simulink library "AEMS_Standard_Library"  (R2016b)
settings: Solver=ode45  StartTime=0.0  StopTime=10.0  RelTol=1e-3
undefined symbols (not defined in the file or in its folder): BkPY, carto, Cbx_extegr, Cbx_lpegrsys, Cbx_portegr, Cnx_bnk_nr_conf, Cnx_cyl_nr_conf, ConfigManagement, configuration_management, Cxx_dcm_io_tmr_end_xxxx, Cxx_dcm_rt_tmr_end, Cxx_DID_xxxx_IO_max, Cxx_DID_xxxx_IO_min, Cxx_egrhsofs, Cxx_vmaniegi, DEM_DEBOUNCE_FREEZE, DEM_DTR_CTL_INVISIBLE, DEM_DTR_CTL_NORMAL, Dem_DtrId2_XXX, Dem_DtrId3_XXX, Dem_DtrId4_XXX, Dem_DtrId5_XXX, Dem_DtrId6_XXX, Dem_DtrId7_XXX, Dem_DtrId8_XXX, Dem_DtrId9_XXX, Dem_DtrId_XXX, Dem_EnableConditionId2_XXX, Dem_EnableConditionId3_XXX, Dem_EnableConditionId4_XXX, Dem_EnableConditionId5_XXX, Dem_EnableConditionId6_XXX, Dem_EnableConditionId7_XXX, Dem_EnableConditionId8_XXX, Dem_EnableConditionId_XXX, Dem_EventId, Dem_EventId2_XXX, Dem_EventId3_XXX, Dem_EventId4_XXX, Dem_EventId5_XXX, Dem_EventId6_XXX, Dem_EventId7_XXX, Dem_EventId8_XXX, Dem_EventId9_XXX, Dem_EventId_Device_Faulttype, Dem_EventId_XXX, DEM_IUMPR_GENERAL_DENOMINATOR, DEM_OPCYC_IGNITION, Dem_RatioId2_XXX, Dem_RatioId3_XXX, Dem_RatioId4_XXX, Dem_RatioId5_XXX, Dem_RatioId6_XXX, Dem_RatioId7_XXX, Dem_RatioId8_XXX, Dem_RatioId_XXX, Dem_StorageConditionId2_XXX, Dem_StorageConditionId3_XXX, Dem_StorageConditionId4_XXX, Dem_StorageConditionId5_XXX ... (+65)
libraries: AEMS_Standard_Library x477, simulink x2
(part 20 of 39)

== system AEMS_Standard_Library/SPECIFIC/AEMS_SUPPLIER_CALL_PHI_MIN_POST ==
  Data Store Read : DataStoreRead  DataStoreName=Supplier_Call_Phi_Min
      settings: AttributesFormatString=<tsample=%<sampleTime>>
  Vxx_fms_phi_min_post : Outport
  wires:
  Data Store Read/1 -> Vxx_fms_phi_min_post/1

== system AEMS_Standard_Library/SPECIFIC/AEMS_SUPPLIER_CALL_QBA_TQI_MAX_LIM ==
  Tqi_raw_wio_qba : Inport
  Tqi_sp : Inport  Port=2
  DataTypeConversion : DataTypeConversion
  Supplier_Call_QBA_TQI_MAX_LIM : DataStoreRead  DataStoreName=Supplier_Call_QBA_TQI_MAX_LIM
      settings: AttributesFormatString=<tsample=%<sampleTime>>
  Terminator : Terminator
  Terminator1 : Terminator
  Tqi_max_lim_qba : Outport  InitialOutput=0
  wires:
  Tqi_sp/1 -> Terminator1/1
  Tqi_raw_wio_qba/1 -> Terminator/1
  Supplier_Call_QBA_TQI_MAX_LIM/1 -> DataTypeConversion/1
  DataTypeConversion/1 -> Tqi_max_lim_qba/1

== system AEMS_Standard_Library/SPECIFIC/AEMS_SUPPLIER_CALL_SEPA_MIN_AFTR ==
  Data Store Read : DataStoreRead  DataStoreName=Supplier_Call_Sepa_Main_Af_Po
      settings: AttributesFormatString=<tsample=%<sampleTime>>
  Vxx_fms_sep_min_aftr : Outport
  wires:
  Data Store Read/1 -> Vxx_fms_sep_min_aftr/1

== system AEMS_Standard_Library/SPECIFIC/AEMS_SUPPLIER_CALL_SEPA_MIN_LPOS ==
  Data Store Read : DataStoreRead  DataStoreName=Supplier_Call_Sepa_Po_Lpost
      settings: AttributesFormatString=<tsample=%<sampleTime>>
  Vxx_fms_sep_min_lpos : Outport
  wires:
  Data Store Read/1 -> Vxx_fms_sep_min_lpos/1

== system AEMS_Standard_Library/SPECIFIC/AEMS_SUPPLIER_CALL_SEPA_MIN_LPOS2_2SL ==
  Data Store Read : DataStoreRead  DataStoreName=Supplier_Call_Sepa_Lpost1_Lpost2
      settings: AttributesFormatString=<tsample=%<sampleTime>>
  Vxx_fms_sep_min_lpos2_2sl : Outport
  wires:
  Data Store Read/1 -> Vxx_fms_sep_min_lpos2_2sl/1

== system AEMS_Standard_Library/SPECIFIC/AEMS_SUPPLIER_CALL_SEPA_MIN_LPOS2_3SL ==
  Data Store Read : DataStoreRead  DataStoreName=Supplier_Call_Sepa_Lpost1_Lpost2
      settings: AttributesFormatString=<tsample=%<sampleTime>>
  Vxx_fms_sep_min_lpos2_3sl : Outport
  wires:
  Data Store Read/1 -> Vxx_fms_sep_min_lpos2_3sl/1

== system AEMS_Standard_Library/SPECIFIC/AEMS_SUPPLIER_CALL_SEPA_MIN_LPOS2_4SL ==
  Data Store Read : DataStoreRead  DataStoreName=Supplier_Call_Sepa_Lpost1_Lpost2
      settings: AttributesFormatString=<tsample=%<sampleTime>>
  Vxx_fms_sep_min_lpos2_4sl : Outport
  wires:
  Data Store Read/1 -> Vxx_fms_sep_min_lpos2_4sl/1

== system AEMS_Standard_Library/SPECIFIC/AEMS_SUPPLIER_CALL_SEPA_MIN_LPOS3_3SL ==
  Data Store Read : DataStoreRead  DataStoreName=Supplier_Call_Sepa_Lpost1_Lpost2
      settings: AttributesFormatString=<tsample=%<sampleTime>>
  Vxx_fms_sep_min_lpos3_3sl : Outport
  wires:
  Data Store Read/1 -> Vxx_fms_sep_min_lpos3_3sl/1

== system AEMS_Standard_Library/SPECIFIC/AEMS_SUPPLIER_CALL_SEPA_MIN_LPOS3_4SL ==
  Data Store Read : DataStoreRead  DataStoreName=Supplier_Call_Sepa_Lpost1_Lpost2
      settings: AttributesFormatString=<tsample=%<sampleTime>>
  Vxx_fms_sep_min_lpos3_4sl : Outport
  wires:
  Data Store Read/1 -> Vxx_fms_sep_min_lpos3_4sl/1

== system AEMS_Standard_Library/SPECIFIC/AEMS_SUPPLIER_CALL_SEPA_MIN_LPOS4_4SL ==
  Data Store Read : DataStoreRead  DataStoreName=Supplier_Call_Sepa_Lpost1_Lpost2
      settings: AttributesFormatString=<tsample=%<sampleTime>>
  Vxx_fms_sep_min_lpos4_4sl : Outport
  wires:
  Data Store Read/1 -> Vxx_fms_sep_min_lpos4_4sl/1

== system AEMS_Standard_Library/SPECIFIC/AEMS_SUPPLIER_CALL_SEPA_MIN_NXT_CYL ==
  Data Store Read : DataStoreRead  DataStoreName=Supplier_Call_Sepa_Lpost_Pinj
      settings: AttributesFormatString=<tsample=%<sampleTime>>
  Vxx_fms_t_min_nxt_cyl : Outport
  wires:
  Data Store Read/1 -> Vxx_fms_t_min_nxt_cyl/1

== system AEMS_Standard_Library/SPECIFIC/AEMS_SUPPLIER_CALL_SEPA_MIN_NXT_CYL_LPOST2 ==
  Data Store Read : DataStoreRead  DataStoreName=Supplier_Call_Sepa_Lpost_Pinj
      settings: AttributesFormatString=<tsample=%<sampleTime>>
  Vxx_fms_t_min_nxt_cyl_lpos2 : Outport
  wires:
  Data Store Read/1 -> Vxx_fms_t_min_nxt_cyl_lpos2/1

== system AEMS_Standard_Library/SPECIFIC/AEMS_SUPPLIER_CALL_SEPA_MIN_NXT_CYL_LPOST3 ==
  Data Store Read : DataStoreRead  DataStoreName=Supplier_Call_Sepa_Lpost_Pinj
      settings: AttributesFormatString=<tsample=%<sampleTime>>
  Vxx_fms_t_min_nxt_cyl_lpos3 : Outport
  wires:
  Data Store Read/1 -> Vxx_fms_t_min_nxt_cyl_lpos3/1

== system AEMS_Standard_Library/SPECIFIC/AEMS_SUPPLIER_CALL_SEPA_MIN_NXT_CYL_LPOST4 ==
  Data Store Read : DataStoreRead  DataStoreName=Supplier_Call_Sepa_Lpost_Pinj
      settings: AttributesFormatString=<tsample=%<sampleTime>>
  Vxx_fms_t_min_nxt_cyl_lpos4 : Outport
  wires:
  Data Store Read/1 -> Vxx_fms_t_min_nxt_cyl_lpos4/1

== system AEMS_Standard_Library/SPECIFIC/AEMS_SUPPLIER_CALL_SEPA_MIN_PINJ1 ==
  Data Store Read : DataStoreRead  DataStoreName=Supplier_Call_Sepa_P1_P2
      settings: AttributesFormatString=<tsample=%<sampleTime>>
  Vxx_fms_tp1_min : Outport
  wires:
  Data Store Read/1 -> Vxx_fms_tp1_min/1

== system AEMS_Standard_Library/SPECIFIC/AEMS_SUPPLIER_CALL_SEPA_MIN_PINJ2 ==
  Data Store Read : DataStoreRead  DataStoreName=Supplier_Call_Sepa_P2_P3
      settings: AttributesFormatString=<tsample=%<sampleTime>>
  Vxx_fms_tp2_min : Outport
  wires:
  Data Store Read/1 -> Vxx_fms_tp2_min/1

== system AEMS_Standard_Library/SPECIFIC/AEMS_SUPPLIER_CALL_SEPA_MIN_PINJ3 ==
  Data Store Read : DataStoreRead  DataStoreName=Supplier_Call_Sepa_P3_P4
      settings: AttributesFormatString=<tsample=%<sampleTime>>
  Vxx_fms_tp3_min : Outport
  wires:
  Data Store Read/1 -> Vxx_fms_tp3_min/1

== system AEMS_Standard_Library/SPECIFIC/AEMS_SUPPLIER_CALL_SEPA_MIN_PINJ4 ==
  Data Store Read : DataStoreRead  DataStoreName=Supplier_Call_Sepa_Pinj_Main
      settings: AttributesFormatString=<tsample=%<sampleTime>>
  Vxx_fms_tp4_min : Outport
  wires:
  Data Store Read/1 -> Vxx_fms_tp4_min/1

== system AEMS_Standard_Library/SPECIFIC/AEMS_SUPPLIER_CALL_SEPA_MIN_POST ==
  Data Store Read : DataStoreRead  DataStoreName=Supplier_Call_Sepa_Main_Af_Po
      settings: AttributesFormatString=<tsample=%<sampleTime>>
  Vxx_fms_sep_min_post : Outport
  wires:
  Data Store Read/1 -> Vxx_fms_sep_min_post/1

== system AEMS_Standard_Library/SPECIFIC/AEMS_SUPPLIER_CALL_SEPERATION_MIN_TIME ==
  note: Each block will be translated into code C by this way:
      | Output=Supplier call API Name(Splitnum);
      | Example for Supplier_Call_Sepa_min_post1, corresponding output variable is
      | Vxx_fms_sep_min_post1= Supplier_Call_Sepa_min_post1(1);
  note: Splitnum
  DataTypeConversion : DataTypeConversion
  Data_Store_Read : DataStoreRead  DataStoreName=Supplier_Call_Sepa_min_post2
  Splitnum : Constant  Value=3  OutDataTypeStr=uint8
  Terminator1 : Terminator
  Vxx_fms_sep_min_post2_3sl : Outport  InitialOutput=0
  wires:
  Splitnum/1 -> Terminator1/1
  Data_Store_Read/1 -> DataTypeConversion/1
  DataTypeConversion/1 -> Vxx_fms_sep_min_post2_3sl/1

== system AEMS_Standard_Library/SPECIFIC/AEMS_SUPPLIER_CALL_TI_MINI_OK_AFTR ==
  Data Store Read : DataStoreRead  DataStoreName=Supplier_call_ti_mini_ok_aftr
      settings: AttributesFormatString=<tsample=%<sampleTime>>
  Vbx_fms_ti_aftr_min_ok : Outport  InitialOutput=0
  wires:
  Data Store Read/1 -> Vbx_fms_ti_aftr_min_ok/1

== system AEMS_Standard_Library/SPECIFIC/AEMS_SUPPLIER_CALL_TI_MINI_OK_LPOS ==
  Data Store Read : DataStoreRead  DataStoreName=Supplier_call_ti_mini_ok_lpos
      settings: AttributesFormatString=<tsample=%<sampleTime>>
  Vbx_fms_ti_lpos_min_ok : Outport  InitialOutput=0
  wires:
  Data Store Read/1 -> Vbx_fms_ti_lpos_min_ok/1

== system AEMS_Standard_Library/SPECIFIC/AEMS_SUPPLIER_CALL_TI_MINI_OK_LPOS1_2SL ==
  Data Store Read : DataStoreRead  DataStoreName=Supplier_call_ti_mini_ok_lpos1
      settings: AttributesFormatString=<tsample=%<sampleTime>>
  Vbx_fms_ti_lpos1_min_ok_2sl : Outport  InitialOutput=0
  wires:
  Data Store Read/1 -> Vbx_fms_ti_lpos1_min_ok_2sl/1

== system AEMS_Standard_Library/SPECIFIC/AEMS_SUPPLIER_CALL_TI_MINI_OK_LPOS1_3SL ==
  Data Store Read : DataStoreRead  DataStoreName=Supplier_call_ti_mini_ok_lpos1
      settings: AttributesFormatString=<tsample=%<sampleTime>>
  Vbx_fms_ti_lpos1_min_ok_3sl : Outport  InitialOutput=0
  wires:
  Data Store Read/1 -> Vbx_fms_ti_lpos1_min_ok_3sl/1

== system AEMS_Standard_Library/SPECIFIC/AEMS_SUPPLIER_CALL_TI_MINI_OK_LPOS1_4SL ==
  Data Store Read : DataStoreRead  DataStoreName=Supplier_call_ti_mini_ok_lpos1
      settings: AttributesFormatString=<tsample=%<sampleTime>>
  Vbx_fms_ti_lpos1_min_ok_4sl : Outport  InitialOutput=0
  wires:
  Data Store Read/1 -> Vbx_fms_ti_lpos1_min_ok_4sl/1

== system AEMS_Standard_Library/SPECIFIC/AEMS_SUPPLIER_CALL_TI_MINI_OK_LPOS2_2SL ==
  Data Store Read : DataStoreRead  DataStoreName=Supplier_call_ti_mini_ok_lpos2
      settings: AttributesFormatString=<tsample=%<sampleTime>>
  Vbx_fms_ti_lpos2_min_ok_2sl : Outport  InitialOutput=0
  wires:
  Data Store Read/1 -> Vbx_fms_ti_lpos2_min_ok_2sl/1

== system AEMS_Standard_Library/SPECIFIC/AEMS_SUPPLIER_CALL_TI_MINI_OK_LPOS2_3SL ==
  Data Store Read : DataStoreRead  DataStoreName=Supplier_call_ti_mini_ok_lpos2
      settings: AttributesFormatString=<tsample=%<sampleTime>>
  Vbx_fms_ti_lpos2_min_ok_3sl : Outport  InitialOutput=0
  wires:
  Data Store Read/1 -> Vbx_fms_ti_lpos2_min_ok_3sl/1

== system AEMS_Standard_Library/SPECIFIC/AEMS_SUPPLIER_CALL_TI_MINI_OK_LPOS2_4SL ==
  Data Store Read : DataStoreRead  DataStoreName=Supplier_call_ti_mini_ok_lpos3
      settings: AttributesFormatString=<tsample=%<sampleTime>>
  Vbx_fms_ti_lpos2_min_ok_4sl : Outport  InitialOutput=0
  wires:
  Data Store Read/1 -> Vbx_fms_ti_lpos2_min_ok_4sl/1

== system AEMS_Standard_Library/SPECIFIC/AEMS_SUPPLIER_CALL_TI_MINI_OK_LPOS3_3SL ==
  Data Store Read : DataStoreRead  DataStoreName=Supplier_call_ti_mini_ok_lpos3
      settings: AttributesFormatString=<tsample=%<sampleTime>>
  Vbx_fms_ti_lpos3_min_ok_3sl : Outport  InitialOutput=0
  wires:
  Data Store Read/1 -> Vbx_fms_ti_lpos3_min_ok_3sl/1

== system AEMS_Standard_Library/SPECIFIC/AEMS_SUPPLIER_CALL_TI_MINI_OK_LPOS3_4SL ==
  Data Store Read : DataStoreRead  DataStoreName=Supplier_call_ti_mini_ok_lpos2
      settings: AttributesFormatString=<tsample=%<sampleTime>>
  Vbx_fms_ti_lpos3_min_ok_4sl : Outport  InitialOutput=0
  wires:
  Data Store Read/1 -> Vbx_fms_ti_lpos3_min_ok_4sl/1

== system AEMS_Standard_Library/SPECIFIC/AEMS_SUPPLIER_CALL_TI_MINI_OK_LPOS4_4SL ==
  Data Store Read : DataStoreRead  DataStoreName=Supplier_call_ti_mini_ok_lpos4
      settings: AttributesFormatString=<tsample=%<sampleTime>>
  Vbx_fms_ti_lpos4_min_ok_4sl : Outport  InitialOutput=0
  wires:
  Data Store Read/1 -> Vbx_fms_ti_lpos4_min_ok_4sl/1

== system AEMS_Standard_Library/SPECIFIC/AEMS_SUPPLIER_CALL_TI_MINI_OK_MAIN ==
  Data Store Read : DataStoreRead  DataStoreName=Supplier_call_ti_mini_ok_main
      settings: AttributesFormatString=<tsample=%<sampleTime>>
  Vbx_fms_ti_main_min_ok : Outport  InitialOutput=0
  wires:
  Data Store Read/1 -> Vbx_fms_ti_main_min_ok/1

== system AEMS_Standard_Library/SPECIFIC/AEMS_SUPPLIER_CALL_TI_MINI_OK_PINJ1 ==
  Data Store Read : DataStoreRead  DataStoreName=Supplier_call_ti_mini_ok_pinj1
      settings: AttributesFormatString=<tsample=%<sampleTime>>
  Vbx_fms_ti_pinj1_min_ok : Outport  InitialOutput=0
  wires:
  Data Store Read/1 -> Vbx_fms_ti_pinj1_min_ok/1

== system AEMS_Standard_Library/SPECIFIC/AEMS_SUPPLIER_CALL_TI_MINI_OK_PINJ2 ==
  Data Store Read : DataStoreRead  DataStoreName=Supplier_call_ti_mini_ok_pinj2
      settings: AttributesFormatString=<tsample=%<sampleTime>>
  Vbx_fms_ti_pinj2_min_ok : Outport  InitialOutput=0
  wires:
  Data Store Read/1 -> Vbx_fms_ti_pinj2_min_ok/1

== system AEMS_Standard_Library/SPECIFIC/AEMS_SUPPLIER_CALL_TI_MINI_OK_PINJ3 ==
  Data Store Read : DataStoreRead  DataStoreName=Supplier_call_ti_mini_ok_pinj3
      settings: AttributesFormatString=<tsample=%<sampleTime>>
  Vbx_fms_ti_pinj3_min_ok : Outport  InitialOutput=0
  wires:
  Data Store Read/1 -> Vbx_fms_ti_pinj3_min_ok/1

== system AEMS_Standard_Library/SPECIFIC/AEMS_SUPPLIER_CALL_TI_MINI_OK_PINJ4 ==
  DataStoreRead : DataStoreRead  DataStoreName=Supplier_call_ti_mini_ok_pinj4
      settings: AttributesFormatString=<tsample=%<sampleTime>>
  Vbx_fms_ti_pinj4_min_ok : Outport  InitialOutput=0
  wires:
  DataStoreRead/1 -> Vbx_fms_ti_pinj4_min_ok/1

== system AEMS_Standard_Library/SPECIFIC/AEMS_SUPPLIER_CALL_TI_MINI_OK_POST ==
  Data Store Read : DataStoreRead  DataStoreName=Supplier_call_ti_mini_ok_post
      settings: AttributesFormatString=<tsample=%<sampleTime>>
  Vbx_fms_ti_post_min_ok : Outport  InitialOutput=0
  wires:
  Data Store Read/1 -> Vbx_fms_ti_post_min_ok/1

== system AEMS_Standard_Library/SPECIFIC/AEMS_SUPPLIER_CALL_TI_MIN_OK ==
  note: Coding information: This block is to call Supplier call API.
      | Each block will be translated into code C by this way:
      | Output=Supplier call API Name(Splitnum);
      | Example for Supplier_Call_Ti_mini_post2_ok, corresponding output variable is
      | Vbx_fms_ti_min_post2_2sl_ok= Supplier_Call_Ti_mini_post2_ok(2);
  note: Splitnum
  DataTypeConversion : DataTypeConversion
  Data_Store_Read : DataStoreRead  DataStoreName=Supplier_Call_Ti_mini_post2_ok
      settings: AttributesFormatString=<tsample=%<sampleTime>>
  Splitnum : Constant  Value=2  OutDataTypeStr=uint8
  Terminator1 : Terminator
  Vbx_fms_ti_min_post2_2sl_ok : Outport  InitialOutput=0
  wires:
  DataTypeConversion/1 -> Vbx_fms_ti_min_post2_2sl_ok/1
  Splitnum/1 -> Terminator1/1
  Data_Store_Read/1 -> DataTypeConversion/1

== system AEMS_Standard_Library/SPECIFIC/AEMS_SlopeSwitchExtern ==
  Switch_Cmd : Inport
  Pos_Slope : Inport  Port=2
  Neg_Slope : Inport  Port=3
  Input : Inport  Port=4
  dT : Inport  Port=5
  Estimate_transition_time : Subsystem
  Product : Product  OutDataTypeStr=Inherit: Inherit via back propagation  RndMeth=Zero
  Product1 : Product  OutDataTypeStr=Inherit: Inherit via back propagation  RndMeth=Zero
  Saturation : Saturate  UpperLimit=1  LowerLimit=0  RndMeth=Zero
      settings: AttributesFormatString=<limits=%<UpperLimit>/%<LowerLimit>>
  Selector : Selector  IndexMode=Zero-based  InputPortWidth=LimitDimInputs  IndexOptions=Index vector (port)  Indices=[1 3]  OutputSizes=1
  Signal_Change_Compute : Subsystem
  Slope_On_Block : Subsystem
  Slope_On_Compute : Subsystem
  Switch2 : Switch  Criteria=u2 ~= 0  RndMeth=Zero  SaturateOnIntegerOverflow=on  InputSameDT=on
      settings: AttributesFormatString=Criteria=%<Criteria>
  UnitDelay1 : UnitDelay  InitialCondition=false  SampleTime=-1
      settings: AttributesFormatString=<initial=%<InitialCondition>>
  UnitDelay2 : UnitDelay  SampleTime=-1
      settings: AttributesFormatString=<initial=%<InitialCondition>>
  Output : Outport
  Slope_On : Outport  Port=2
  Rem_Transition_Time : Outport  Port=3
  wires:
  Neg_Slope/1 -> Product1/2, Estimate_transition_time/4(Neg_Slope)
  Selector/1 -> Switch2/3, Estimate_transition_time/1(Input), Slope_On_Block/2(Input)
  Pos_Slope/1 -> Product/2, Estimate_transition_time/3(Pos_Slope)
  Slope_On_Block/1(Output_Not_Equals_Input) -> UnitDelay1/1
  Switch2/1 -> UnitDelay2/1, Estimate_transition_time/2(Output), Output/1
  Slope_On_Compute/1(Slope_On) -> Switch2/2, Slope_On_Block/Enable, Slope_On/1  "Slope_On"
  Slope_On_Block/2(Output) -> Switch2/1
  UnitDelay1/1 -> Slope_On_Compute/2(Output_Not_Equals_Input)
  Switch_Cmd/1 -> Saturation/1
  UnitDelay2/1 -> Slope_On_Block/5(Prev_Output)
  Product/1 -> Slope_On_Block/3(Pos_Slope)
  Product1/1 -> Slope_On_Block/4(Neg_Slope)
  Signal_Change_Compute/1(Signal_Change) -> Slope_On_Compute/1(Signal_Change), Slope_On_Block/1(Signal_Change)
  dT/1 -> Product/1, Product1/1
  Estimate_transition_time/1(Rem_Transition_Time) -> Rem_Transition_Time/1
  Input/1 -> Selector/1
  Saturation/1 -> Selector/2, Signal_Change_Compute/1(Switch_Cmd)

== system AEMS_Standard_Library/SPECIFIC/AEMS_UL_INTERP ==
  input_of_ratio_1 : Inport
      settings: AttributesFormatString=<tsample=%<sampleTime>>
  interpolate_ratio : Inport  Port=2
      settings: AttributesFormatString=<tsample=%<sampleTime>>
  input_of_ratio_0 : Inport  Port=3
      settings: AttributesFormatString=<tsample=%<sampleTime>>
  Constant1 : Constant  OutDataTypeStr=Inherit: Inherit via back propagation
  Product : Product  OutDataTypeStr=Inherit: Inherit via back propagation  RndMeth=Zero
  Product1 : Product  OutDataTypeStr=Inherit: Inherit via back propagation  RndMeth=Zero
  Saturation : Saturate  UpperLimit=1  LowerLimit=0
      settings: AttributesFormatString=<limits=%<upperlimit> / %<lowerlimit>>
  Sum : Sum  Inputs=-+  SaturateOnIntegerOverflow=on  InputSameDT=on
  Sum1 : Sum  SaturateOnIntegerOverflow=on  InputSameDT=on
  output : Outport
  wires:
  Sum1/1 -> output/1
  Constant1/1 -> Sum/2
  input_of_ratio_0/1 -> Product1/2
  Product1/1 -> Sum1/2
  Product/1 -> Sum1/1
  Sum/1 -> Product1/1
  interpolate_ratio/1 -> Saturation/1
  input_of_ratio_1/1 -> Product/1
  Saturation/1 -> Product/2, Sum/1

== system AEMS_Standard_Library/SUB/AEMS_CONVERT_BUFFER_TO_FLP ==
  note: Scalar Value in FXP
  note: Value_FLP
  note: Conversion from FXP to FLP
      |
      | Data converted from FXP to FLP using Resolution and Offset of variable DID
  note: ERRORCode: Retrun status of Error Code
      |
      | Data written by DCM in array form and converted to
      | a scalar by multiplied by factor [1 2^8 2^16 2^24] depend on size of DID
  Buffer : Inport
  Chart1 : Stateflow chart  TreatAsAtomicUnit=on
  Constant : Constant  Value=DID_Datatype  OutDataTypeStr=uint8
  Data Type Conversion : DataTypeConversion
  Mux : Mux  Inputs=3
  Offset : Constant  Value=offset  OutDataTypeStr=Inherit: Inherit via back propagation
  Product1 : Product  OutDataTypeStr=Inherit: Inherit via back propagation  RndMeth=Zero
  Resol : Constant  Value=Resol  OutDataTypeStr=Inherit: Inherit via back propagation
  Sum1 : Sum  OutDataTypeStr=Inherit: Inherit via back propagation  RndMeth=Zero  InputSameDT=on
  Terminator : Terminator
  Value_float : Outport
  wires:
  Mux/1 -> Terminator/1
  Sum1/1 -> Value_float/1, Mux/1
  Product1/1 -> Sum1/1
  Resol/1 -> Product1/2, Mux/3
  Offset/1 -> Sum1/2, Mux/2
  Data Type Conversion/1 -> Product1/1
  Buffer/1 -> Chart1/2(Input_Buff)
  Chart1/1(Fxp_Scalar_Value) -> Data Type Conversion/1
  Constant/1 -> Chart1/1(DataType)

== system AEMS_Standard_Library/SUB/AEMS_CONVERT_BYTE_TO_FLP ==
  note: ERRORCode: Retrun status of Error Code
      |
      | Data written by DCM in array form and converted to
      | a scalar by multiplied by factor [1 2^8 2^16 2^24] depend on size of DID
  note: Conversion from FXP to FLP
      |
      | Data converted from FXP to FLP using Resolution and Offset of variable DID
  note: Value_FLP
  note: Scalar Value in FXP
  Input : Inport
  Chart1 : Stateflow chart  TreatAsAtomicUnit=on
  Constant : Constant  Value=DID_Datatype  OutDataTypeStr=uint8
  Data Type Conversion : DataTypeConversion
  Mux : Mux  Inputs=3
  Offset : Constant  Value=offset  OutDataTypeStr=Inherit: Inherit via back propagation
  Product1 : Product  OutDataTypeStr=Inherit: Inherit via back propagation  RndMeth=Zero
  Resol : Constant  Value=Resol  OutDataTypeStr=Inherit: Inherit via back propagation
  Sum1 : Sum  OutDataTypeStr=Inherit: Inherit via back propagation  RndMeth=Zero  InputSameDT=on
  Terminator : Terminator
  Value_float : Outport
  wires:
  Constant/1 -> Chart1/1(DataType)
  Chart1/1(Fxp_Scalar_Value) -> Data Type Conversion/1
  Input/1 -> Chart1/2(Input)
  Data Type Conversion/1 -> Product1/1
  Offset/1 -> Mux/2, Sum1/2
  Resol/1 -> Mux/3, Product1/2
  Product1/1 -> Sum1/1
  Sum1/1 -> Mux/1, Value_float/1
  Mux/1 -> Terminator/1

== system AEMS_Standard_Library/SUB/AEMS_DEM_COUNTERBASEDDEBOUNCE ==
  conditionfulfilled : Inport
  prefailed : Inport  Port=2
  prepassed : Inport  Port=3
  reseteventdebounce : Inport  Port=4
  DemDebounceBehavior : Inport  Port=5
  DemCounterFailedThreshold : Inport  Port=6
  DemCounterIncrementStepSize : Inport  Port=7
  DemCounterJumpUp : Inport  Port=8
  DemCounterJumpUpValue : Inport  Port=9
  DemCounterPassedThreshold : Inport  Port=10
  DemCounterDecrementStepSize : Inport  Port=11
  DemCounterJumpDown : Inport  Port=12
  DemCounterJumpDownValue : Inport  Port=13
  Counter_Debounce : Subsystem
  Dem_SetEventStatus_Call : Subsystem  TreatAsAtomicUnit=on
  debouncevalue : Outport
  failed : Outport  Port=2
  passed : Outport  Port=3
  wires:
  conditionfulfilled/1 -> Counter_Debounce/1(conditionfulfilled)
  Counter_Debounce/3(passed) -> passed/1
  Counter_Debounce/2(failed) -> failed/1
  reseteventdebounce/1 -> Counter_Debounce/13(reseteventdebounce)
  DemCounterJumpDownValue/1 -> Counter_Debounce/12(jumpdownvalue_with_prepassed)
  DemCounterJumpDown/1 -> Counter_Debounce/11(jumpdown_activation_with_prepassed)
  DemCounterDecrementStepSize/1 -> Counter_Debounce/10(decrementstepsize_for_prepassed)
  DemCounterPassedThreshold/1 -> Counter_Debounce/9(passedthreshold)
  DemCounterJumpUpValue/1 -> Counter_Debounce/8(jumpupvalue_with_prefailed)
  DemCounterJumpUp/1 -> Counter_Debounce/7(jumpup_activation_with_prefailed)
  DemCounterIncrementStepSize/1 -> Counter_Debounce/6(incrementstepsize_for_prefailed)
  Counter_Debounce/5(eventstatus) -> Dem_SetEventStatus_Call/1(event_status)
  DemCounterFailedThreshold/1 -> Counter_Debounce/5(failedthreshold)
  DemDebounceBehavior/1 -> Counter_Debounce/4(behavior)
  prefailed/1 -> Counter_Debounce/2(prefailed)
  prepassed/1 -> Counter_Debounce/3(prepassed)
  Counter_Debounce/1(debouncevalue) -> debouncevalue/1
  Counter_Debounce/4(call_seteventstatus) -> Dem_SetEventStatus_Call/Enable

== system AEMS_Standard_Library/SUB/AEMS_DEM_COUNTER_BASED_DEBOUNCE_1D ==
  note: DemDebounceBehavior
  flag_set : Inport
  conditionfulfilled : Inport  Port=2
  prefailed : Inport  Port=3
  prepassed : Inport  Port=4
  reseteventdebounce : Inport  Port=5
  AEMS_DEM_COUNTER_BASED_DEBOUNCE_CALL : Subsystem
  DemCounterDecrementStepSize : Constant  Value=DemCounterDecrementStepSize
  DemCounterFailedThreshold : Constant  Value=DemCounterFailedThreshold
  DemCounterIncrementStepSize : Constant  Value=DemCounterIncrementStepSize
  DemCounterJumpDown : Constant  Value=DemCounterJumpDown
  DemCounterJumpDownValue : Constant  Value=DemCounterJumpDownValue
  DemCounterJumpUp : Constant  Value=DemCounterJumpUp
  DemCounterJumpUpValue : Constant  Value=DemCounterJumpUpValue
  DemCounterPassedThreshold : Constant  Value=DemCounterPassedThreshold
  DemDebounceBehavior : Constant  Value=0  OutDataTypeStr=uint8
  debouncevalue : Outport
  failed : Outport  Port=2
  passed : Outport  Port=3
  wires:
  flag_set/1 -> AEMS_DEM_COUNTER_BASED_DEBOUNCE_CALL/Enable
  AEMS_DEM_COUNTER_BASED_DEBOUNCE_CALL/3(passed) -> passed/1
  AEMS_DEM_COUNTER_BASED_DEBOUNCE_CALL/2(failed) -> failed/1
  AEMS_DEM_COUNTER_BASED_DEBOUNCE_CALL/1(debouncevalue) -> debouncevalue/1
  DemCounterJumpDownValue/1 -> AEMS_DEM_COUNTER_BASED_DEBOUNCE_CALL/13(DemCounterJumpDownValue)  "jumpupvalue_with_prefailed"
  DemCounterJumpDown/1 -> AEMS_DEM_COUNTER_BASED_DEBOUNCE_CALL/12(DemCounterJumpDown)  "jumpdown_activation_with_prepassed"
  DemCounterDecrementStepSize/1 -> AEMS_DEM_COUNTER_BASED_DEBOUNCE_CALL/11(DemCounterDecrementStepSize)  "decrementstepsize_for_prepassed"
  DemCounterPassedThreshold/1 -> AEMS_DEM_COUNTER_BASED_DEBOUNCE_CALL/10(DemCounterPassedThreshold)  "passedthreshold"
  DemCounterJumpUpValue/1 -> AEMS_DEM_COUNTER_BASED_DEBOUNCE_CALL/9(DemCounterJumpUpValue)  "jumpupvalue_with_prefailed"
  DemCounterJumpUp/1 -> AEMS_DEM_COUNTER_BASED_DEBOUNCE_CALL/8(DemCounterJumpUp)  "jumpup_activation_with_prefailed"
  DemCounterIncrementStepSize/1 -> AEMS_DEM_COUNTER_BASED_DEBOUNCE_CALL/7(DemCounterIncrementStepSize)  "incrementstepsize_for_prefailed"
  DemCounterFailedThreshold/1 -> AEMS_DEM_COUNTER_BASED_DEBOUNCE_CALL/6(DemCounterFailedThreshold)  "failedthreshold"
  DemDebounceBehavior/1 -> AEMS_DEM_COUNTER_BASED_DEBOUNCE_CALL/5(DemDebounceBehavior)  "behavior"
  reseteventdebounce/1 -> AEMS_DEM_COUNTER_BASED_DEBOUNCE_CALL/4(reseteventdebounce)  "reseteventdebounce"
  prepassed/1 -> AEMS_DEM_COUNTER_BASED_DEBOUNCE_CALL/3(prepassed)  "prepassed"
  prefailed/1 -> AEMS_DEM_COUNTER_BASED_DEBOUNCE_CALL/2(prefailed)  "prefailed"
  conditionfulfilled/1 -> AEMS_DEM_COUNTER_BASED_DEBOUNCE_CALL/1(conditionfulfilled)  "conditionfulfilled"

== system AEMS_Standard_Library/SUB/AEMS_DEM_COUNTER_BASED_DEBOUNCE_2D ==
  note: DemDebounceBehavior
  flag_set : Inport
  conditionfulfilled : Inport  Port=2
  prefailed : Inport  Port=3
  prepassed : Inport  Port=4
  reseteventdebounce : Inport  Port=5
  AEMS_DEM_COUNTER_BASED_DEBOUNCE_CALL1 : Subsystem
  AEMS_DEM_COUNTER_BASED_DEBOUNCE_CALL2 : Subsystem
  DemCounterDecrementStepSize : Constant  Value=DemCounterDecrementStepSize
  DemCounterFailedThreshold : Constant  Value=DemCounterFailedThreshold
  DemCounterIncrementStepSize : Constant  Value=DemCounterIncrementStepSize
  DemCounterJumpDown : Constant  Value=DemCounterJumpDown
  DemCounterJumpDownValue : Constant  Value=DemCounterJumpDownValue
  DemCounterJumpUp : Constant  Value=DemCounterJumpUp
  DemCounterJumpUpValue : Constant  Value=DemCounterJumpUpValue
  DemCounterPassedThreshold : Constant  Value=DemCounterPassedThreshold
  DemDebounceBehavior : Constant  Value=[0,0]  OutDataTypeStr=uint8
  Demux{,1..4} (5 alike) : Demux  Outputs=[1,1]
  Demux{5..13} (9 alike) : Demux  Outputs=2
  Mux : Mux  Inputs=2
  Mux1 : Mux  Inputs=2
  Mux2 : Mux  Inputs=2
  debouncevalue : Outport
  failed : Outport  Port=2
  passed : Outport  Port=3
  wires:
  AEMS_DEM_COUNTER_BASED_DEBOUNCE_CALL2/3(passed) -> Mux/2
  AEMS_DEM_COUNTER_BASED_DEBOUNCE_CALL2/2(failed) -> Mux2/2
  AEMS_DEM_COUNTER_BASED_DEBOUNCE_CALL2/1(debouncevalue) -> Mux1/2
  AEMS_DEM_COUNTER_BASED_DEBOUNCE_CALL1/3(passed) -> Mux/1
  AEMS_DEM_COUNTER_BASED_DEBOUNCE_CALL1/2(failed) -> Mux2/1
  AEMS_DEM_COUNTER_BASED_DEBOUNCE_CALL1/1(debouncevalue) -> Mux1/1
  Mux2/1 -> failed/1
  Mux1/1 -> debouncevalue/1
  Mux/1 -> passed/1
  Demux7/1 -> AEMS_DEM_COUNTER_BASED_DEBOUNCE_CALL1/13(DemCounterJumpDownValue)
  Demux6/1 -> AEMS_DEM_COUNTER_BASED_DEBOUNCE_CALL1/12(DemCounterJumpDown)
  Demux5/1 -> AEMS_DEM_COUNTER_BASED_DEBOUNCE_CALL1/11(DemCounterDecrementStepSize)
  Demux10/1 -> AEMS_DEM_COUNTER_BASED_DEBOUNCE_CALL1/10(DemCounterPassedThreshold)
  Demux9/1 -> AEMS_DEM_COUNTER_BASED_DEBOUNCE_CALL1/9(DemCounterJumpUpValue)
  Demux8/1 -> AEMS_DEM_COUNTER_BASED_DEBOUNCE_CALL1/8(DemCounterJumpUp)
  Demux13/1 -> AEMS_DEM_COUNTER_BASED_DEBOUNCE_CALL1/7(DemCounterIncrementStepSize)
  Demux12/1 -> AEMS_DEM_COUNTER_BASED_DEBOUNCE_CALL1/6(DemCounterFailedThreshold)
  Demux11/1 -> AEMS_DEM_COUNTER_BASED_DEBOUNCE_CALL1/5(DemDebounceBehavior)
  Demux4/1 -> AEMS_DEM_COUNTER_BASED_DEBOUNCE_CALL1/4(reseteventdebounce)
  Demux3/1 -> AEMS_DEM_COUNTER_BASED_DEBOUNCE_CALL1/3(prepassed)
  Demux2/1 -> AEMS_DEM_COUNTER_BASED_DEBOUNCE_CALL1/2(prefailed)
  Demux1/1 -> AEMS_DEM_COUNTER_BASED_DEBOUNCE_CALL1/1(conditionfulfilled)
  Demux/1 -> AEMS_DEM_COUNTER_BASED_DEBOUNCE_CALL1/Enable
  Demux/2 -> AEMS_DEM_COUNTER_BASED_DEBOUNCE_CALL2/Enable
  Demux1/2 -> AEMS_DEM_COUNTER_BASED_DEBOUNCE_CALL2/1(conditionfulfilled)
  Demux2/2 -> AEMS_DEM_COUNTER_BASED_DEBOUNCE_CALL2/2(prefailed)
  Demux3/2 -> AEMS_DEM_COUNTER_BASED_DEBOUNCE_CALL2/3(prepassed)
  Demux4/2 -> AEMS_DEM_COUNTER_BASED_DEBOUNCE_CALL2/4(reseteventdebounce)
  Demux11/2 -> AEMS_DEM_COUNTER_BASED_DEBOUNCE_CALL2/5(DemDebounceBehavior)
  Demux12/2 -> AEMS_DEM_COUNTER_BASED_DEBOUNCE_CALL2/6(DemCounterFailedThreshold)
  Demux13/2 -> AEMS_DEM_COUNTER_BASED_DEBOUNCE_CALL2/7(DemCounterIncrementStepSize)
  Demux8/2 -> AEMS_DEM_COUNTER_BASED_DEBOUNCE_CALL2/8(DemCounterJumpUp)
  Demux9/2 -> AEMS_DEM_COUNTER_BASED_DEBOUNCE_CALL2/9(DemCounterJumpUpValue)
  Demux10/2 -> AEMS_DEM_COUNTER_BASED_DEBOUNCE_CALL2/10(DemCounterPassedThreshold)
  Demux5/2 -> AEMS_DEM_COUNTER_BASED_DEBOUNCE_CALL2/11(DemCounterDecrementStepSize)
  Demux6/2 -> AEMS_DEM_COUNTER_BASED_DEBOUNCE_CALL2/12(DemCounterJumpDown)
  Demux7/2 -> AEMS_DEM_COUNTER_BASED_DEBOUNCE_CALL2/13(DemCounterJumpDownValue)
  DemCounterIncrementStepSize/1 -> Demux13/1  "incrementstepsize_for_prefailed"
  DemCounterFailedThreshold/1 -> Demux12/1  "failedthreshold"
  DemDebounceBehavior/1 -> Demux11/1  "behavior"
  DemCounterPassedThreshold/1 -> Demux10/1  "passedthreshold"
  DemCounterJumpUpValue/1 -> Demux9/1  "jumpupvalue_with_prefailed"
  DemCounterJumpUp/1 -> Demux8/1  "jumpup_activation_with_prefailed"
  DemCounterJumpDownValue/1 -> Demux7/1  "jumpupvalue_with_prefailed"
  DemCounterJumpDown/1 -> Demux6/1  "jumpdown_activation_with_prepassed"
  DemCounterDecrementStepSize/1 -> Demux5/1  "decrementstepsize_for_prepassed"
  reseteventdebounce/1 -> Demux4/1  "reseteventdebounce"
  prepassed/1 -> Demux3/1  "prepassed"
  prefailed/1 -> Demux2/1  "prefailed"
  conditionfulfilled/1 -> Demux1/1  "conditionfulfilled"
  flag_set/1 -> Demux/1

== system AEMS_Standard_Library/SUB/AEMS_DEM_COUNTER_BASED_DEBOUNCE_3D ==
  note: DemDebounceBehavior
  flag_set : Inport
  conditionfulfilled : Inport  Port=2
  prefailed : Inport  Port=3
  prepassed : Inport  Port=4
  reseteventdebounce : Inport  Port=5
  AEMS_DEM_COUNTER_BASED_DEBOUNCE_CALL1 : Subsystem
  AEMS_DEM_COUNTER_BASED_DEBOUNCE_CALL2 : Subsystem
  AEMS_DEM_COUNTER_BASED_DEBOUNCE_CALL3 : Subsystem
  DemCounterDecrementStepSize : Constant  Value=DemCounterDecrementStepSize
  DemCounterFailedThreshold : Constant  Value=DemCounterFailedThreshold
  DemCounterIncrementStepSize : Constant  Value=DemCounterIncrementStepSize
  DemCounterJumpDown : Constant  Value=DemCounterJumpDown
  DemCounterJumpDownValue : Constant  Value=DemCounterJumpDownValue
  DemCounterJumpUp : Constant  Value=DemCounterJumpUp
  DemCounterJumpUpValue : Constant  Value=DemCounterJumpUpValue
  DemCounterPassedThreshold : Constant  Value=DemCounterPassedThreshold
  DemDebounceBehavior : Constant  Value=[0,0,0]  OutDataTypeStr=uint8
  Demux{,1..13} (14 alike) : Demux  Outputs=3
  Mux : Mux  Inputs=3
  Mux1 : Mux  Inputs=3
  Mux2 : Mux  Inputs=3
  debouncevalue : Outport
  failed : Outport  Port=2
  passed : Outport  Port=3
  wires:
  AEMS_DEM_COUNTER_BASED_DEBOUNCE_CALL3/3(passed) -> Mux/3
  AEMS_DEM_COUNTER_BASED_DEBOUNCE_CALL3/2(failed) -> Mux2/3
  AEMS_DEM_COUNTER_BASED_DEBOUNCE_CALL3/1(debouncevalue) -> Mux1/3
  Demux7/3 -> AEMS_DEM_COUNTER_BASED_DEBOUNCE_CALL3/13(DemCounterJumpDownValue)
  Demux6/3 -> AEMS_DEM_COUNTER_BASED_DEBOUNCE_CALL3/12(DemCounterJumpDown)
  Demux5/3 -> AEMS_DEM_COUNTER_BASED_DEBOUNCE_CALL3/11(DemCounterDecrementStepSize)
  Demux10/3 -> AEMS_DEM_COUNTER_BASED_DEBOUNCE_CALL3/10(DemCounterPassedThreshold)
  Demux9/3 -> AEMS_DEM_COUNTER_BASED_DEBOUNCE_CALL3/9(DemCounterJumpUpValue)
  Demux8/3 -> AEMS_DEM_COUNTER_BASED_DEBOUNCE_CALL3/8(DemCounterJumpUp)
  Demux13/3 -> AEMS_DEM_COUNTER_BASED_DEBOUNCE_CALL3/7(DemCounterIncrementStepSize)
  Demux12/3 -> AEMS_DEM_COUNTER_BASED_DEBOUNCE_CALL3/6(DemCounterFailedThreshold)
  Demux11/3 -> AEMS_DEM_COUNTER_BASED_DEBOUNCE_CALL3/5(DemDebounceBehavior)
  Demux4/3 -> AEMS_DEM_COUNTER_BASED_DEBOUNCE_CALL3/4(reseteventdebounce)
  Demux3/3 -> AEMS_DEM_COUNTER_BASED_DEBOUNCE_CALL3/3(prepassed)
  Demux2/3 -> AEMS_DEM_COUNTER_BASED_DEBOUNCE_CALL3/2(prefailed)
  Demux1/3 -> AEMS_DEM_COUNTER_BASED_DEBOUNCE_CALL3/1(conditionfulfilled)
  Demux/3 -> AEMS_DEM_COUNTER_BASED_DEBOUNCE_CALL3/Enable
  AEMS_DEM_COUNTER_BASED_DEBOUNCE_CALL2/3(passed) -> Mux/2
  AEMS_DEM_COUNTER_BASED_DEBOUNCE_CALL2/2(failed) -> Mux2/2
  AEMS_DEM_COUNTER_BASED_DEBOUNCE_CALL2/1(debouncevalue) -> Mux1/2
  AEMS_DEM_COUNTER_BASED_DEBOUNCE_CALL1/3(passed) -> Mux/1
  AEMS_DEM_COUNTER_BASED_DEBOUNCE_CALL1/2(failed) -> Mux2/1
  AEMS_DEM_COUNTER_BASED_DEBOUNCE_CALL1/1(debouncevalue) -> Mux1/1
  Mux2/1 -> failed/1
  Mux1/1 -> debouncevalue/1
  Mux/1 -> passed/1
  Demux7/1 -> AEMS_DEM_COUNTER_BASED_DEBOUNCE_CALL1/13(DemCounterJumpDownValue)
  Demux6/1 -> AEMS_DEM_COUNTER_BASED_DEBOUNCE_CALL1/12(DemCounterJumpDown)
  Demux5/1 -> AEMS_DEM_COUNTER_BASED_DEBOUNCE_CALL1/11(DemCounterDecrementStepSize)
  Demux10/1 -> AEMS_DEM_COUNTER_BASED_DEBOUNCE_CALL1/10(DemCounterPassedThreshold)
  Demux9/1 -> AEMS_DEM_COUNTER_BASED_DEBOUNCE_CALL1/9(DemCounterJumpUpValue)
  Demux8/1 -> AEMS_DEM_COUNTER_BASED_DEBOUNCE_CALL1/8(DemCounterJumpUp)
  Demux13/1 -> AEMS_DEM_COUNTER_BASED_DEBOUNCE_CALL1/7(DemCounterIncrementStepSize)
  Demux12/1 -> AEMS_DEM_COUNTER_BASED_DEBOUNCE_CALL1/6(DemCounterFailedThreshold)
  Demux11/1 -> AEMS_DEM_COUNTER_BASED_DEBOUNCE_CALL1/5(DemDebounceBehavior)
  Demux4/1 -> AEMS_DEM_COUNTER_BASED_DEBOUNCE_CALL1/4(reseteventdebounce)
  Demux3/1 -> AEMS_DEM_COUNTER_BASED_DEBOUNCE_CALL1/3(prepassed)
  Demux2/1 -> AEMS_DEM_COUNTER_BASED_DEBOUNCE_CALL1/2(prefailed)
  Demux1/1 -> AEMS_DEM_COUNTER_BASED_DEBOUNCE_CALL1/1(conditionfulfilled)
  Demux/1 -> AEMS_DEM_COUNTER_BASED_DEBOUNCE_CALL1/Enable
  Demux/2 -> AEMS_DEM_COUNTER_BASED_DEBOUNCE_CALL2/Enable
  Demux1/2 -> AEMS_DEM_COUNTER_BASED_DEBOUNCE_CALL2/1(conditionfulfilled)
  Demux2/2 -> AEMS_DEM_COUNTER_BASED_DEBOUNCE_CALL2/2(prefailed)
  Demux3/2 -> AEMS_DEM_COUNTER_BASED_DEBOUNCE_CALL2/3(prepassed)
  Demux4/2 -> AEMS_DEM_COUNTER_BASED_DEBOUNCE_CALL2/4(reseteventdebounce)
  Demux11/2 -> AEMS_DEM_COUNTER_BASED_DEBOUNCE_CALL2/5(DemDebounceBehavior)
  Demux12/2 -> AEMS_DEM_COUNTER_BASED_DEBOUNCE_CALL2/6(DemCounterFailedThreshold)
  Demux13/2 -> AEMS_DEM_COUNTER_BASED_DEBOUNCE_CALL2/7(DemCounterIncrementStepSize)
  Demux8/2 -> AEMS_DEM_COUNTER_BASED_DEBOUNCE_CALL2/8(DemCounterJumpUp)
  Demux9/2 -> AEMS_DEM_COUNTER_BASED_DEBOUNCE_CALL2/9(DemCounterJumpUpValue)
  Demux10/2 -> AEMS_DEM_COUNTER_BASED_DEBOUNCE_CALL2/10(DemCounterPassedThreshold)
  Demux5/2 -> AEMS_DEM_COUNTER_BASED_DEBOUNCE_CALL2/11(DemCounterDecrementStepSize)
  Demux6/2 -> AEMS_DEM_COUNTER_BASED_DEBOUNCE_CALL2/12(DemCounterJumpDown)
  Demux7/2 -> AEMS_DEM_COUNTER_BASED_DEBOUNCE_CALL2/13(DemCounterJumpDownValue)
  DemCounterIncrementStepSize/1 -> Demux13/1  "incrementstepsize_for_prefailed"
  DemCounterFailedThreshold/1 -> Demux12/1  "failedthreshold"
  DemDebounceBehavior/1 -> Demux11/1  "behavior"
  DemCounterPassedThreshold/1 -> Demux10/1  "passedthreshold"
  DemCounterJumpUpValue/1 -> Demux9/1  "jumpupvalue_with_prefailed"
  DemCounterJumpUp/1 -> Demux8/1  "jumpup_activation_with_prefailed"
  DemCounterJumpDownValue/1 -> Demux7/1  "jumpupvalue_with_prefailed"
  DemCounterJumpDown/1 -> Demux6/1  "jumpdown_activation_with_prepassed"
  DemCounterDecrementStepSize/1 -> Demux5/1  "decrementstepsize_for_prepassed"
  reseteventdebounce/1 -> Demux4/1  "reseteventdebounce"
  prepassed/1 -> Demux3/1  "prepassed"
  prefailed/1 -> Demux2/1  "prefailed"
  conditionfulfilled/1 -> Demux1/1  "conditionfulfilled"
  flag_set/1 -> Demux/1

== system AEMS_Standard_Library/SUB/AEMS_DEM_COUNTER_BASED_DEBOUNCE_4D ==
  note: DemDebounceBehavior
  flag_set : Inport
  conditionfulfilled : Inport  Port=2
  prefailed : Inport  Port=3
  prepassed : Inport  Port=4
  reseteventdebounce : Inport  Port=5
  AEMS_DEM_COUNTER_BASED_DEBOUNCE_CALL1 : Subsystem
  AEMS_DEM_COUNTER_BASED_DEBOUNCE_CALL2 : Subsystem
  AEMS_DEM_COUNTER_BASED_DEBOUNCE_CALL3 : Subsystem
  AEMS_DEM_COUNTER_BASED_DEBOUNCE_CALL4 : Subsystem
  DemCounterDecrementStepSize : Constant  Value=DemCounterDecrementStepSize
  DemCounterFailedThreshold : Constant  Value=DemCounterFailedThreshold
  DemCounterIncrementStepSize : Constant  Value=DemCounterIncrementStepSize
  DemCounterJumpDown : Constant  Value=DemCounterJumpDown
  DemCounterJumpDownValue : Constant  Value=DemCounterJumpDownValue
  DemCounterJumpUp : Constant  Value=DemCounterJumpUp
  DemCounterJumpUpValue : Constant  Value=DemCounterJumpUpValue
  DemCounterPassedThreshold : Constant  Value=DemCounterPassedThreshold
  DemDebounceBehavior : Constant  Value=[0,0,0,0]  OutDataTypeStr=uint8
  Demux{,1..13} (14 alike) : Demux
  Mux : Mux
  Mux1 : Mux
  Mux2 : Mux
  debouncevalue : Outport
  failed : Outport  Port=2
  passed : Outport  Port=3
  wires:
  AEMS_DEM_COUNTER_BASED_DEBOUNCE_CALL4/3(passed) -> Mux/4
  AEMS_DEM_COUNTER_BASED_DEBOUNCE_CALL4/2(failed) -> Mux2/4
  AEMS_DEM_COUNTER_BASED_DEBOUNCE_CALL4/1(debouncevalue) -> Mux1/4
  Demux7/4 -> AEMS_DEM_COUNTER_BASED_DEBOUNCE_CALL4/13(DemCounterJumpDownValue)
  Demux6/4 -> AEMS_DEM_COUNTER_BASED_DEBOUNCE_CALL4/12(DemCounterJumpDown)
  Demux5/4 -> AEMS_DEM_COUNTER_BASED_DEBOUNCE_CALL4/11(DemCounterDecrementStepSize)
  Demux10/4 -> AEMS_DEM_COUNTER_BASED_DEBOUNCE_CALL4/10(DemCounterPassedThreshold)
  Demux9/4 -> AEMS_DEM_COUNTER_BASED_DEBOUNCE_CALL4/9(DemCounterJumpUpValue)
  Demux8/4 -> AEMS_DEM_COUNTER_BASED_DEBOUNCE_CALL4/8(DemCounterJumpUp)
  Demux13/4 -> AEMS_DEM_COUNTER_BASED_DEBOUNCE_CALL4/7(DemCounterIncrementStepSize)
  Demux12/4 -> AEMS_DEM_COUNTER_BASED_DEBOUNCE_CALL4/6(DemCounterFailedThreshold)
  Demux11/4 -> AEMS_DEM_COUNTER_BASED_DEBOUNCE_CALL4/5(DemDebounceBehavior)
  Demux4/4 -> AEMS_DEM_COUNTER_BASED_DEBOUNCE_CALL4/4(reseteventdebounce)
  Demux3/4 -> AEMS_DEM_COUNTER_BASED_DEBOUNCE_CALL4/3(prepassed)
  Demux2/4 -> AEMS_DEM_COUNTER_BASED_DEBOUNCE_CALL4/2(prefailed)
  Demux1/4 -> AEMS_DEM_COUNTER_BASED_DEBOUNCE_CALL4/1(conditionfulfilled)
  Demux/4 -> AEMS_DEM_COUNTER_BASED_DEBOUNCE_CALL4/Enable
  flag_set/1 -> Demux/1
  conditionfulfilled/1 -> Demux1/1  "conditionfulfilled"
  prefailed/1 -> Demux2/1  "prefailed"
  prepassed/1 -> Demux3/1  "prepassed"
  reseteventdebounce/1 -> Demux4/1  "reseteventdebounce"
  DemCounterDecrementStepSize/1 -> Demux5/1  "decrementstepsize_for_prepassed"
  DemCounterJumpDown/1 -> Demux6/1  "jumpdown_activation_with_prepassed"
  DemCounterJumpDownValue/1 -> Demux7/1  "jumpupvalue_with_prefailed"
  DemCounterJumpUp/1 -> Demux8/1  "jumpup_activation_with_prefailed"
  DemCounterJumpUpValue/1 -> Demux9/1  "jumpupvalue_with_prefailed"
  DemCounterPassedThreshold/1 -> Demux10/1  "passedthreshold"
  DemDebounceBehavior/1 -> Demux11/1  "behavior"
  DemCounterFailedThreshold/1 -> Demux12/1  "failedthreshold"
  DemCounterIncrementStepSize/1 -> Demux13/1  "incrementstepsize_for_prefailed"
  Demux7/2 -> AEMS_DEM_COUNTER_BASED_DEBOUNCE_CALL2/13(DemCounterJumpDownValue)
  Demux6/2 -> AEMS_DEM_COUNTER_BASED_DEBOUNCE_CALL2/12(DemCounterJumpDown)
  Demux5/2 -> AEMS_DEM_COUNTER_BASED_DEBOUNCE_CALL2/11(DemCounterDecrementStepSize)
  Demux10/2 -> AEMS_DEM_COUNTER_BASED_DEBOUNCE_CALL2/10(DemCounterPassedThreshold)
  Demux9/2 -> AEMS_DEM_COUNTER_BASED_DEBOUNCE_CALL2/9(DemCounterJumpUpValue)
  Demux8/2 -> AEMS_DEM_COUNTER_BASED_DEBOUNCE_CALL2/8(DemCounterJumpUp)
  Demux13/2 -> AEMS_DEM_COUNTER_BASED_DEBOUNCE_CALL2/7(DemCounterIncrementStepSize)
  Demux12/2 -> AEMS_DEM_COUNTER_BASED_DEBOUNCE_CALL2/6(DemCounterFailedThreshold)
  Demux11/2 -> AEMS_DEM_COUNTER_BASED_DEBOUNCE_CALL2/5(DemDebounceBehavior)
  Demux4/2 -> AEMS_DEM_COUNTER_BASED_DEBOUNCE_CALL2/4(reseteventdebounce)
  Demux3/2 -> AEMS_DEM_COUNTER_BASED_DEBOUNCE_CALL2/3(prepassed)
  Demux2/2 -> AEMS_DEM_COUNTER_BASED_DEBOUNCE_CALL2/2(prefailed)
  Demux1/2 -> AEMS_DEM_COUNTER_BASED_DEBOUNCE_CALL2/1(conditionfulfilled)
  Demux/2 -> AEMS_DEM_COUNTER_BASED_DEBOUNCE_CALL2/Enable
  Demux/1 -> AEMS_DEM_COUNTER_BASED_DEBOUNCE_CALL1/Enable
  Demux1/1 -> AEMS_DEM_COUNTER_BASED_DEBOUNCE_CALL1/1(conditionfulfilled)
  Demux2/1 -> AEMS_DEM_COUNTER_BASED_DEBOUNCE_CALL1/2(prefailed)
  Demux3/1 -> AEMS_DEM_COUNTER_BASED_DEBOUNCE_CALL1/3(prepassed)
  Demux4/1 -> AEMS_DEM_COUNTER_BASED_DEBOUNCE_CALL1/4(reseteventdebounce)
  Demux11/1 -> AEMS_DEM_COUNTER_BASED_DEBOUNCE_CALL1/5(DemDebounceBehavior)
  Demux12/1 -> AEMS_DEM_COUNTER_BASED_DEBOUNCE_CALL1/6(DemCounterFailedThreshold)
  Demux13/1 -> AEMS_DEM_COUNTER_BASED_DEBOUNCE_CALL1/7(DemCounterIncrementStepSize)
  Demux8/1 -> AEMS_DEM_COUNTER_BASED_DEBOUNCE_CALL1/8(DemCounterJumpUp)
  Demux9/1 -> AEMS_DEM_COUNTER_BASED_DEBOUNCE_CALL1/9(DemCounterJumpUpValue)
  Demux10/1 -> AEMS_DEM_COUNTER_BASED_DEBOUNCE_CALL1/10(DemCounterPassedThreshold)
  Demux5/1 -> AEMS_DEM_COUNTER_BASED_DEBOUNCE_CALL1/11(DemCounterDecrementStepSize)
  Demux6/1 -> AEMS_DEM_COUNTER_BASED_DEBOUNCE_CALL1/12(DemCounterJumpDown)
  Demux7/1 -> AEMS_DEM_COUNTER_BASED_DEBOUNCE_CALL1/13(DemCounterJumpDownValue)
  Mux/1 -> passed/1
  Mux1/1 -> debouncevalue/1
  Mux2/1 -> failed/1
  AEMS_DEM_COUNTER_BASED_DEBOUNCE_CALL1/1(debouncevalue) -> Mux1/1
  AEMS_DEM_COUNTER_BASED_DEBOUNCE_CALL1/2(failed) -> Mux2/1
  AEMS_DEM_COUNTER_BASED_DEBOUNCE_CALL1/3(passed) -> Mux/1
  AEMS_DEM_COUNTER_BASED_DEBOUNCE_CALL2/1(debouncevalue) -> Mux1/2
  AEMS_DEM_COUNTER_BASED_DEBOUNCE_CALL2/2(failed) -> Mux2/2
  AEMS_DEM_COUNTER_BASED_DEBOUNCE_CALL2/3(passed) -> Mux/2
  Demux/3 -> AEMS_DEM_COUNTER_BASED_DEBOUNCE_CALL3/Enable
  Demux1/3 -> AEMS_DEM_COUNTER_BASED_DEBOUNCE_CALL3/1(conditionfulfilled)
  Demux2/3 -> AEMS_DEM_COUNTER_BASED_DEBOUNCE_CALL3/2(prefailed)
  Demux3/3 -> AEMS_DEM_COUNTER_BASED_DEBOUNCE_CALL3/3(prepassed)
  Demux4/3 -> AEMS_DEM_COUNTER_BASED_DEBOUNCE_CALL3/4(reseteventdebounce)
  Demux11/3 -> AEMS_DEM_COUNTER_BASED_DEBOUNCE_CALL3/5(DemDebounceBehavior)
  Demux12/3 -> AEMS_DEM_COUNTER_BASED_DEBOUNCE_CALL3/6(DemCounterFailedThreshold)
  Demux13/3 -> AEMS_DEM_COUNTER_BASED_DEBOUNCE_CALL3/7(DemCounterIncrementStepSize)
  Demux8/3 -> AEMS_DEM_COUNTER_BASED_DEBOUNCE_CALL3/8(DemCounterJumpUp)
  Demux9/3 -> AEMS_DEM_COUNTER_BASED_DEBOUNCE_CALL3/9(DemCounterJumpUpValue)
  Demux10/3 -> AEMS_DEM_COUNTER_BASED_DEBOUNCE_CALL3/10(DemCounterPassedThreshold)
  Demux5/3 -> AEMS_DEM_COUNTER_BASED_DEBOUNCE_CALL3/11(DemCounterDecrementStepSize)
  Demux6/3 -> AEMS_DEM_COUNTER_BASED_DEBOUNCE_CALL3/12(DemCounterJumpDown)
  Demux7/3 -> AEMS_DEM_COUNTER_BASED_DEBOUNCE_CALL3/13(DemCounterJumpDownValue)
  AEMS_DEM_COUNTER_BASED_DEBOUNCE_CALL3/1(debouncevalue) -> Mux1/3
  AEMS_DEM_COUNTER_BASED_DEBOUNCE_CALL3/2(failed) -> Mux2/3
  AEMS_DEM_COUNTER_BASED_DEBOUNCE_CALL3/3(passed) -> Mux/3
